simulink model "lab10"  (R2021b)
settings: Solver=VariableStepAuto  StartTime=0.0  StopTime=10.0  RelTol=1e-3
libraries: commrandsrc3 x1, commsynccomp2 x1
settings Model: LastModifiedBy=qwert123

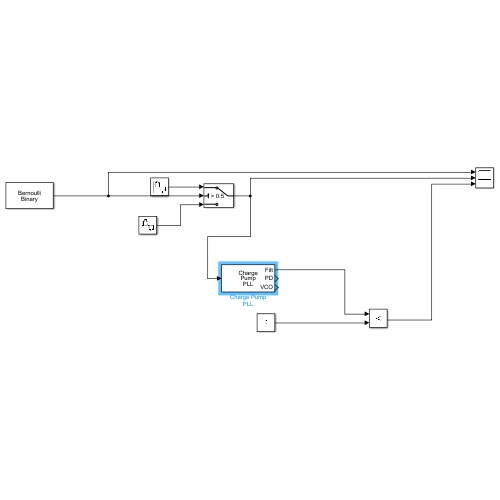
[thumbnail: Simulink's stored preview of the top-level diagram]
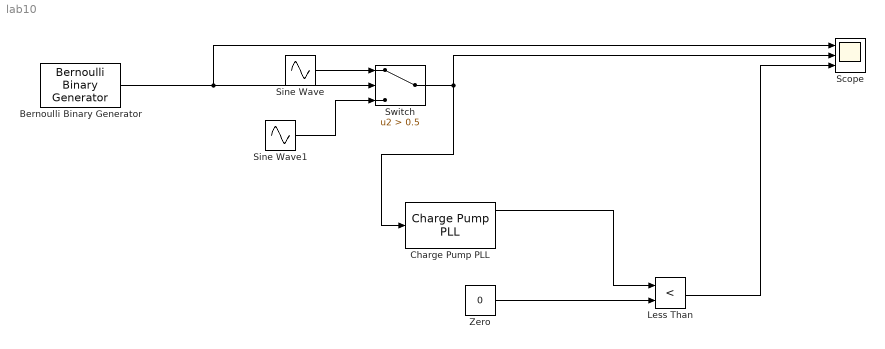
== system lab10 ==
  Bernoulli Binary Generator : commrandsrc3/Bernoulli Binary Generator  ProbabilityOfZero=0.5  SeedSource=Auto  Seed=0  SampleTime=1  SamplesPerFrame=1  OutputDataType=double  SimulateUsing=Interpreted execution
  Charge Pump PLL : commsynccomp2/Charge Pump PLL  Fn=[2*pi*1]  Fd="[1   2*pi*1]"  Kvco=4  Fc=10  Ph=0  Ac=1
      settings: SourceProductBaseCode=CM
  Less Than : RelationalOperator  Operator=<  OutDataTypeStr=boolean  RndMeth=Simplest
  Scope : Scope  NumInputPorts=3
  Sine Wave : Sin  Frequency=2*pi*4  SampleTime=0.01
  Sine Wave1 : Sin  Frequency=2*pi*12  SampleTime=0.01
  Switch : Switch  Criteria=u2 > Threshold  Threshold=0.5
  Zero : Constant  Value=0  OutDataTypeStr=Inherit: Inherit via back propagation
  wires:
  Sine Wave/1 -> Switch/1
  Bernoulli Binary Generator/1 -> Scope/1, Switch/2
  Sine Wave1/1 -> Switch/3
  Switch/1 -> Charge Pump PLL/1, Scope/2
  Charge Pump PLL/1 -> Less Than/1
  Zero/1 -> Less Than/2
  Less Than/1 -> Scope/3
